simulink model "mpcprueba1"  (R2025a)
settings: Solver=FixedStepAuto  StartTime=0.0  StopTime=inf  FixedStep=0.015  RelTol=1e-3  EnableMultiTasking=on
libraries: px4Sensorslib x2, px4Peripheralslib x1
settings Model: PacingRate=0.790000  ExtModeTrigDuration=10  Creator=The MathWorks, Inc.  LastModifiedBy=aero
settings SolverCC: AlgebraicLoopSolver=TrustRegion  PositivePriorityOrder=on  AutoInsertRateTranBlk=on  MaxZcPerStep=1.0
settings OptimizationCC: EnhancedBackFolding=on  PassReuseOutputArgsAs=Individual arguments  MaxStackSize=64  OptimizeBlockOrder=speed  DifferentSizesBufferReuse=on  OptimizationCustomize=off  EfficientTunableParamExpr=on
settings DebuggingCC: ParameterPrecisionLossMsg=none  ParameterTunabilityLossMsg=error  UnconnectedInputMsg=warning  UnconnectedOutputMsg=warning  UnconnectedLineMsg=warning  SubsystemReferenceDiagnosticForUnitTest=warning  ArithmeticOperatorsInVariantConditions=warning
settings HardwareCC: ProdBitPerPointer=32.0  ProdBitPerSizeT=32.0  ProdBitPerPtrDiffT=32.0  ProdLargestAtomicInteger=Long  ProdLargestAtomicFloat=Double  ProdWordSize=32.0  ProdLongLongMode=on  ProdHWDeviceType=ARM Compatible->ARM Cortex
settings ModelReferenceCC: EnableRefExpFcnMdlSchedulingChecks=on
settings SFSimCC: MATLABDynamicMemAlloc=off  SimTargetLang=C++  SimDLTargetLibrary=mkl-dnn
settings RTWCC: SystemTargetFile=ert.tlc  HardwareBoard=PX4 Pixhawk 6c  TLCOptions="-aInlineSetEventsForThisBaseRateFcn=TLC_FALSE -aSuppressMultiTaskScheduler=TLC_FALSE  -aRateBasedStepFcn=0"  TemplateMakefile=ert_default_tmf  GenerateReport=on  Toolchain=GNU Tools for PX4 Autopilots  IncludeHyperlinkInReport=on  LaunchReport=on  TargetLang=C++  GenerateTraceInfo=on  GenerateTraceReport=on  GenerateTraceReportSl=on  GenerateTraceReportSf=on  GenerateTraceReportEml=on  GPUComputeCapability=3.5  DLArmComputeVersion=19.05  Description=Embedded Coder
settings CodeAppCC: ForceParamTrailComments=on  IgnoreCustomStorageClasses=off  OperatorAnnotations=on  SimulinkDataObjDesc=on  SFDataObjDesc=on  InsertBlockDesc=on
settings ERTTargetCC: ExtModeTransport=3.0  ExtModeStaticAllocSize=1024.0  InlinedParameterPlacement=Hierarchical

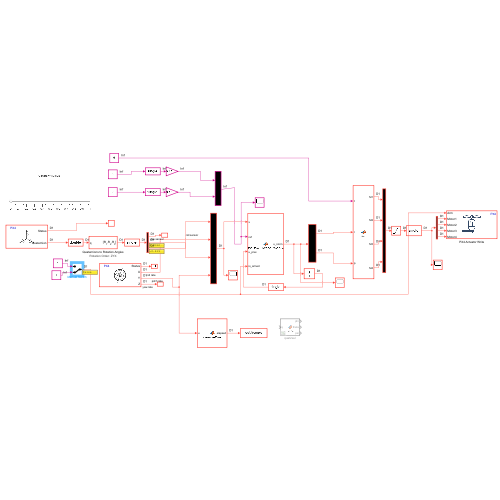
[thumbnail: Simulink's stored preview of the top-level diagram]
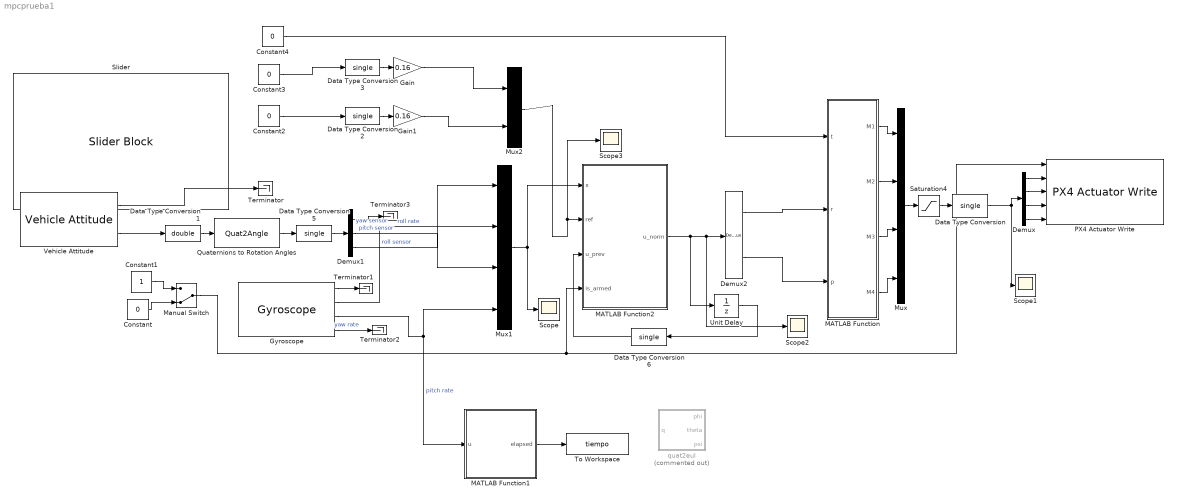
== system mpcprueba1 ==
  Constant : Constant  Value=0  OutDataTypeStr=boolean
  Constant1 : Constant  OutDataTypeStr=boolean
  Constant2 : Constant  Value=0
  Constant3 : Constant  Value=0
  Constant4 : Constant  Value=0
  Data Type Conversion{,2..3,5..6} (5 alike) : DataTypeConversion  OutDataTypeStr=single  SaturateOnIntegerOverflow=off  RndMeth=Floor
  Data Type Conversion1 : DataTypeConversion  OutDataTypeStr=double  SaturateOnIntegerOverflow=off  RndMeth=Floor
  Demux : Demux
  Demux1 : Demux  Outputs=3
  Demux2 : Demux  Outputs=2
  Gain : Gain  Gain=0.16
  Gain1 : Gain  Gain=0.16
  Gyroscope : px4Sensorslib/Gyroscope  uorbTimeStamp=off  BlockingMode=off  BlockTimeout=1e-3  sampleTime=0.015
  MATLAB Function : MATLAB Function  TreatAsAtomicUnit=on
  MATLAB Function1 : MATLAB Function  TreatAsAtomicUnit=on
  MATLAB Function2 : MATLAB Function  TreatAsAtomicUnit=on
  Manual Switch : ManualSwitch  CurrentSetting=0
  Mux : Mux
  Mux1 : Mux
  Mux2 : Mux  Inputs=2
  PX4 Actuator Write : px4Peripheralslib/PX4 Actuator Write  Motor1Enable=on  Motor2Enable=on  Motor3Enable=on  Motor4Enable=on  Motor5Enable=off  Motor6Enable=off  Motor7Enable=off  Motor8Enable=off  Motor9Enable=off  Motor10Enable=off  Motor11Enable=off  Motor12Enable=off  IsMotorArray=off  Servo1Enable=off  Servo2Enable=off  Servo3Enable=off  Servo4Enable=off  Servo5Enable=off  Servo6Enable=off  Servo7Enable=off  Servo8Enable=off  IsServoArray=off
  Quaternions to Rotation Angles : Quat2Angle
      settings: AttributesFormatString=Rotation Order: %<rotationOrder>
  Saturation4 : Saturate  UpperLimit=1  LowerLimit=0
  Scope{,1..3} (4 alike) : Scope
      Scope settings: ActiveDisplayYMinimum=-1.9109067916870117  ActiveDisplayYMaximum=3.8255419731140137
      Scope1 settings: ActiveDisplayYMinimum=-1.9221124811650505  ActiveDisplayYMaximum=2.19156354528468  DataLoggingVariableName=ScopeData3
      Scope2 settings: ActiveDisplayYMinimum=-0.36091258117677238  ActiveDisplayYMaximum=1.3022961290231061
      Scope3 settings: ActiveDisplayYMinimum=-1  ActiveDisplayYMaximum=1  DataLoggingVariableName=ScopeData2
  Slider : SliderBlock  ScaleMax=1
  Terminator{,1..3} (4 alike) : Terminator
  To Workspace : ToWorkspace  VariableName=tiempo  SaveFormat=Timeseries  SampleTime=-1
  Unit Delay : UnitDelay  SampleTime=-1  HasFrameUpgradeWarning=on
  Vehicle Attitude : px4Sensorslib/Vehicle Attitude  rollRate=off  pitchRate=off  yawRate=off  quaternion=on  uorbTimeStamp=off  BlockingMode=off  BlockTimeout=0.001  sampleTime=0.015
  quat2eul : MATLAB Function  Commented=on  TreatAsAtomicUnit=on
  wires:
  Manual Switch/1 -> MATLAB Function2/4(is_armed), PX4 Actuator Write/1
  Mux1/1 -> Scope/1, MATLAB Function2/1(x)
  Mux2/1 -> Scope3/1, MATLAB Function2/2(ref)
  Vehicle Attitude/1 -> Terminator/1
  Vehicle Attitude/2 -> Data Type Conversion1/1
  Demux2/2 -> MATLAB Function/3(p)
  Mux/1 -> Saturation4/1
  Gain1/1 -> Mux2/2
  Constant3/1 -> Data Type Conversion3/1
  Gyroscope/2 -> Mux1/2  "roll rate"
  Data Type Conversion3/1 -> Gain/1
  Data Type Conversion5/1 -> Demux1/1
  MATLAB Function1/1(elapsed) -> To Workspace/1
  Demux/2 -> PX4 Actuator Write/3
  Gain/1 -> Mux2/1
  Data Type Conversion/1 -> Demux/1, Scope1/1
  Demux1/3 -> Mux1/1  "roll sensor"
  MATLAB Function2/1(u_norm) -> Unit Delay/1, Scope2/1, Demux2/1
  Constant1/1 -> Manual Switch/1
  Demux1/2 -> Mux1/3  "pitch sensor"
  Gyroscope/3 -> Mux1/4, MATLAB Function1/1(u)  "pitch rate"
  Saturation4/1 -> Data Type Conversion/1
  Demux/1 -> PX4 Actuator Write/2
  MATLAB Function/1(M1) -> Mux/1
  Quaternions to Rotation Angles/1 -> Data Type Conversion5/1
  Constant/1 -> Manual Switch/2
  Demux/3 -> PX4 Actuator Write/4
  Demux/4 -> PX4 Actuator Write/5
  Demux2/1 -> MATLAB Function/2(r)
  Gyroscope/1 -> Terminator1/1
  Data Type Conversion6/1 -> MATLAB Function2/3(u_prev)
  Data Type Conversion2/1 -> Gain1/1
  Constant4/1 -> MATLAB Function/1(t)
  Unit Delay/1 -> Data Type Conversion6/1
  Data Type Conversion1/1 -> Quaternions to Rotation Angles/1
  Constant2/1 -> Data Type Conversion2/1
  Gyroscope/4 -> Terminator2/1  "yaw rate"
  Demux1/1 -> Terminator3/1  "yaw sensor"
  MATLAB Function/2(M2) -> Mux/2
  MATLAB Function/3(M3) -> Mux/3
  MATLAB Function/4(M4) -> Mux/4

== matlab function mpcprueba1/MATLAB Function1 ==
  data: u input; elapsed output
function elapsed = measureTime(u)
% u: entrada dummy para forzar ejecución por step
%#codegen

elapsed = 0.0;   %  tipo fijo (double escalar)

coder.extrinsic('tic','toc')

persistent tStart
if isempty(tStart)
    tStart = tic;
end

elapsed = toc(tStart);
tStart = tic;

== matlab function mpcprueba1/MATLAB Function ==
  data: t input; M1 output; r input; p input; M2 output; M3 output; M4 output
function [M1,M2,M3,M4]  = fcn(t,r, p)
M1 = t - 0.707107*r + 0.707107*p;
M2 = t + 0.707107*r - 0.707107*p;
M3 = t + 0.707107*r + 0.707107*p;
M4 = t - 0.707107*r - 0.707107*p;

== matlab function mpcprueba1/MATLAB Function2 ==
  data: x input; u_norm output; ref input; u_prev input; is_armed input
function u_norm = MPC_Eolo_V2806_SoftStart(x, ref, u_prev, is_armed)
    persistent Ad Bd Cd F Phi H_inv x_old Nc Np m n_aug x_filt Q_total
    
    Ts = single(0.015);  
    Np_val = 10; 
    Nc_val = 2; 
    n_s = 4; 
    m_in = 2; 
    q_out = 2; 
    
    if isempty(Ad)
        Np = Np_val; Nc = Nc_val;
        m = m_in; q = q_out;
        Ixx = single(0.048); Iyy = single(0.048); 
        
        Ac = single([0 1 0 0; 0 0 0 0; 0 0 1 0; 0 0 0 0]);
        Bc = single([0 0; 1.2/Ixx 0; 0 0; 0 1.2/Iyy]); % Ganancia ligeramente reducida para suavidad
        Cd = single([1 0 0 0; 0 0 1 0]); 
        
        Ad = eye(4, 'single') + Ac * Ts;
        Ad(2,2) = single(0.85); Ad(4,4) = single(0.85); % Más amortiguamiento
        Bd = Bc * Ts;
        
        n_aug = n_s + q;
        A_aug = [Ad, zeros(n_s, q, 'single'); Cd*Ad, eye(q, 'single') * single(0.5)]; 
        B_aug = [Bd; Cd*Bd];
        C_aug = [zeros(q, n_s, 'single'), eye(q, 'single')];
        
        F = zeros(Np*q, n_aug, 'single');
        Phi = zeros(Np*q, Nc*m, 'single');
        
        temp_A = A_aug;
        for i = 1:Np
            F((i-1)*q+1:i*q, :) = C_aug * temp_A;
            for j = 1:Nc
                if i >= j
                    Phi((i-1)*q+1:i*q, (j-1)*m+1:j*m) = C_aug * (A_aug^(i-j)) * B_aug;
                end
            end
            temp_A = temp_A * A_aug;
        end
        
        Q_total = zeros(Np*q, Np*q, 'single');
        Q_sub = single(diag([400, 400])); % Bajamos Q para evitar el inicio brusco
        for i = 1:Np; Q_total((i-1)*q+1:i*q, (i-1)*q+1:i*q) = Q_sub; end
        
        Rw = eye(Nc*m, 'single') * single(3000.0); % Rw alto para cambios lentos
        H_inv = inv(Phi' * Q_total * Phi + Rw);
        
        x_old = zeros(4, 1, 'single'); 
        x_filt = zeros(4, 1, 'single');
    end

    if isempty(Q_total)
        u_norm = single([0.0; 0.0]); return;
    end

    % --- ESTADO DESARMADO / INICIO DESDE 0 ---
    if is_armed < single(0.5)
        u_norm = single([0.0; 0.0]); 
        x_old = single(x); 
        x_filt = single(x);
        return;
    end

    x_s = single(0.8) * x_filt + single(0.2) * single(x); % Filtro más fuerte
    x_filt = x_s;
    
    error_vec = [x_s(1)-ref(1); x_s(3)-ref(2)];
    delta_x = x_s - x_old;
    x_aug = [delta_x; error_vec];
    
    Rs = zeros(Np_val*q_out, 1, 'single'); 
    dU = -H_inv * (Phi' * Q_total * (Rs - F * x_aug));
    
    % --- LIMITADOR DE RAMPA (Soft-Start Dinámico) ---
    % No permitimos que el motor cambie más de 0.02 (2%) por paso de 15ms
    max_step = single(0.02);
    dU_limited = [max(min(dU(1), max_step), -max_step);
                  max(min(dU(2), max_step), -max_step)];
    
    u_raw = single(u_prev) + dU_limited;
    
    % Saturación: de 0 a 0.85
    u_norm = [max(min(u_raw(1), single(0.85)), single(0.0));
              max(min(u_raw(2), single(0.85)), single(0.0))];
    
    x_old = x_s;
end

== matlab function mpcprueba1/quat2eul ==
  data: q input; phi output; theta output; psi output
function [phi,theta,psi] = quat2eul(q)

% Quaternion conversion to Euler angles based on the PX4 Firmware v1.10.2
% release.

phi = atan2(2*(q(1)*q(2) + q(3)* q(4)), q(1)^2 - q(2)^2 - q(3)^2 + q(4)^2);
theta = asin(-2*(q(2)*q(4) - q(1)*q(3)));
psi = atan2(2*(q(2)*q(3) + q(1)* q(4)), q(1)^2 + q(2)^2 - q(3)^2 - q(4)^2);
end
